simulink model "Comparison_Modulation_Techniques"  (R2021a)
settings: Solver=VariableStepAuto  StartTime=0.0  StopTime=10.0  RelTol=1e-3
libraries: commchan3 x4, commdigbbndpm3 x4, commsink2 x4, commrandsrc3 x3, commdigbbndfm2 x2, commdigbbndam3 x2, dspsrcs4 x1, dspquant2 x1
settings Model: Creator=Bharat Gunhalkar  LastModifiedBy=Bharat Gunhalkar

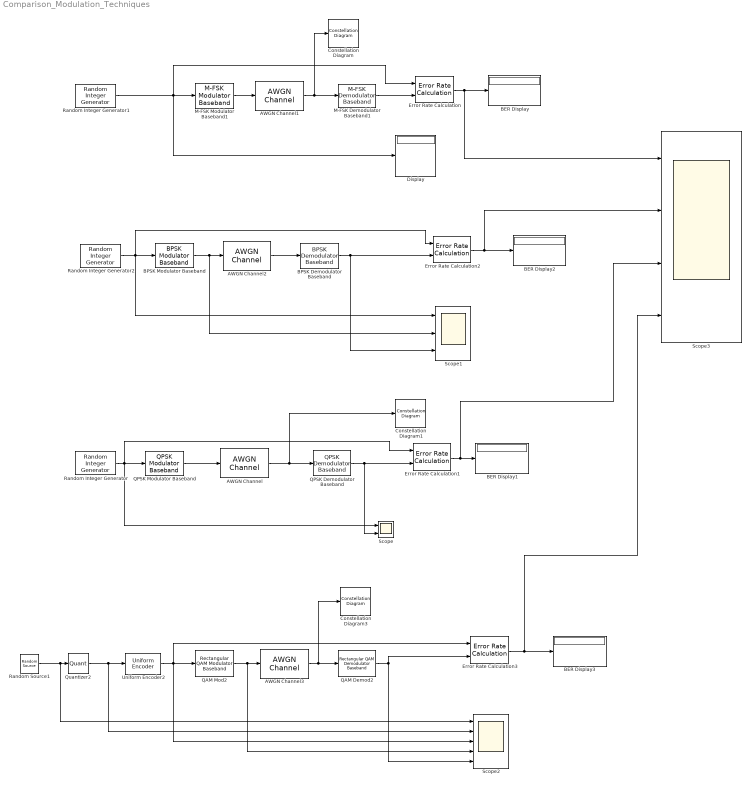
== system Comparison_Modulation_Techniques ==
  AWGN Channel : commchan3/AWGN Channel  InputProcessing=Columns as channels (frame based)  seed=67  noiseMode="Signal to noise ratio  (Eb/No)"  EbNodB=1  EsNodB=10  SNRdB=10  bitsPerSym=2  Ps=1  Tsym=1  variance=1
  AWGN Channel1 : commchan3/AWGN Channel  InputProcessing=Columns as channels (frame based)  seed=67  noiseMode="Signal to noise ratio  (Eb/No)"  EbNodB=1  EsNodB=10  SNRdB=10  bitsPerSym=1  Ps=1  Tsym=1  variance=1
  AWGN Channel2 : commchan3/AWGN Channel  InputProcessing=Columns as channels (frame based)  seed=67  noiseMode="Signal to noise ratio  (Eb/No)"  EbNodB=1  EsNodB=10  SNRdB=10  bitsPerSym=1  Ps=1  Tsym=1  variance=1
  AWGN Channel3 : commchan3/AWGN Channel  InputProcessing=Columns as channels (frame based)  seed=67  noiseMode="Signal to noise ratio  (Eb/No)"  EbNodB=1  EsNodB=10  SNRdB=10  bitsPerSym=1  Ps=1  Tsym=1  variance=1
  BER Display{,1..3} (4 alike) : Display
  BPSK Demodulator Baseband : commdigbbndpm3/BPSK Demodulator Baseband  DecType=Hard decision  VarSource=Dialog  Variance=1  Ph=0  outDtype=Inherit via internal rule  derotateFactorWordLen=16  derotateFactorDataTypeStr=Inherit: Same word length as input  derotateFactorLastDataTypeStr=Inherit: Same word length as input
  BPSK Modulator Baseband : commdigbbndpm3/BPSK Modulator Baseband  Ph=0  outDtype=double  outWordLen=16  outUDDataType=sfix(16)  outFracLenMode=Best precision  outFracLen=15  outDataTypeStr=double  outLastDataTypeStr=double
  Constellation Diagram : ConstellationDiagram
  Constellation Diagram1 : ConstellationDiagram
  Constellation Diagram3 : ConstellationDiagram
  Display : Display
  Error Rate Calculation{,1..3} (4 alike) : commsink2/Error Rate Calculation  N=0  st_delay=0  cp_mode=Entire frame  subframe=[]  PMode=Port  WsName=ErrorVec  RsMode2=off  stop=off  numErr=100  maxBits=1e6
  M-FSK Demodulator Baseband1 : commdigbbndfm2/M-FSK Demodulator Baseband  M=8  OutType=Integer  Dec=Gray  freqSep=6  numSamp=17  RateOptions=Enforce single-rate processing  outDataType=double
      settings: SourceProductBaseCode=CM
  M-FSK Modulator Baseband1 : commdigbbndfm2/M-FSK Modulator Baseband  M=8  InType=Integer  Enc=Gray  freqSep=6  phaseType=Continuous  numSamp=17  RateOptions=Enforce single-rate processing  outDataType=double
  QAM Demod2 : commdigbbndam3/Rectangular QAM Demodulator Baseband  M=16  OutType=Integer  DecType=Hard decision  VarSource=Dialog  Variance=1  Dec=Gray  Mapping=[0:15]  PowType=Min. distance between symbols  MinDist=2  AvgPow=1  PeakPow=1  Ph=0  outDtype1=Inherit via internal rule  outDtype2=Inherit via internal rule  derotateFactorWordLen=16  derotateFactorDataTypeStr=Inherit: Same word length as input  derotateFactorLastDataTypeStr=Inherit: Same word length as input  denormFactorWordLen=16  denormFactorDataTypeStr=Inherit: Same word length as input  denormFactorLastDataTypeStr=Inherit: Same word length as input  prodOutWordLen=32  prodOutOverflowMode=Wrap  prodOutRoundingMode=Floor  prodOutOvFlMode=off  prodOutOvFlModeLastStrValue=off  sumWordLen=32
  QAM Mod2 : commdigbbndam3/Rectangular QAM Modulator Baseband  M=16  InType=Integer  Enc=Gray  Mapping=[0:15]  PowType=Min. distance between symbols  MinDist=2  AvgPow=1  PeakPow=1  Ph=0  outDtype=double  outWordLen=16  outUDDataType=sfix(16)  outFracLenMode=Best precision  outFracLen=15  outDataTypeStr=double  outLastDataTypeStr=double
  QPSK Demodulator Baseband : commdigbbndpm3/QPSK Demodulator Baseband  OutType=Integer  DecType=Hard decision  VarSource=Dialog  Variance=1  Dec=Gray  Ph=pi/4  outDtype1=Inherit via internal rule  outDtype2=Inherit via internal rule  derotateFactorWordLen=16  derotateFactorDataTypeStr=Inherit: Same word length as input  derotateFactorLastDataTypeStr=Inherit: Same word length as input
  QPSK Modulator Baseband : commdigbbndpm3/QPSK Modulator Baseband  InType=Integer  Enc=Gray  Ph=pi/4  outDtype=double  outWordLen=16  outUDDataType=sfix(16)  outFracLenMode=Best precision  outFracLen=15  outDataTypeStr=double  outLastDataTypeStr=double
  Quantizer2 : Quantizer  QuantizationInterval=0.25  LinearizeAsGain=off
  Random Source1 : dspsrcs4/Random Source  SrcType=Uniform  NormMethod=Ziggurat  CltLength=12  MinVal=0  MaxVal=1  MeanVal=0  VarVal=1  RepMode=Not repeatable  rawSeed=1  IsInherit=off  SampMode=Discrete  SampTime=0.1  SampFrame=1  DataType=Single  OutComplex=Real  OutputFrames=off
  Random Integer Generator : commrandsrc3/Random Integer Generator  SetSize=4  SeedSource=Auto  Seed=0  SampleTime=1  SamplesPerFrame=1  OutputDataType=double  SimulateUsing=Interpreted execution
  Random Integer Generator1 : commrandsrc3/Random Integer Generator  SetSize=8  SeedSource=Auto  Seed=0  SampleTime=1  SamplesPerFrame=100  OutputDataType=double  SimulateUsing=Interpreted execution
  Random Integer Generator2 : commrandsrc3/Random Integer Generator  SetSize=2  SeedSource=Auto  Seed=0  SampleTime=0.1  SamplesPerFrame=1  OutputDataType=double  SimulateUsing=Interpreted execution
  Scope : Scope  NumInputPorts=2
  Scope1 : Scope  NumInputPorts=3
  Scope2 : Scope  NumInputPorts=5
  Scope3 : Scope  NumInputPorts=4
  Uniform Encoder2 : dspquant2/Uniform Encoder  peak=1  bits=4  otype=Unsigned integer
  wires:
  M-FSK Modulator Baseband1/1 -> AWGN Channel1/1
  Error Rate Calculation/1 -> Scope3/1, BER Display/1
  M-FSK Demodulator Baseband1/1 -> Error Rate Calculation/2
  AWGN Channel1/1 -> M-FSK Demodulator Baseband1/1, Constellation Diagram/1
  Random Integer Generator1/1 -> Display/1, Error Rate Calculation/1, M-FSK Modulator Baseband1/1
  AWGN Channel2/1 -> BPSK Demodulator Baseband/1
  Error Rate Calculation2/1 -> Scope3/2, BER Display2/1
  BPSK Demodulator Baseband/1 -> Error Rate Calculation2/2, Scope1/3
  Random Integer Generator2/1 -> Scope1/1, BPSK Modulator Baseband/1, Error Rate Calculation2/1
  BPSK Modulator Baseband/1 -> Scope1/2, AWGN Channel2/1
  Error Rate Calculation1/1 -> Scope3/3, BER Display1/1
  QPSK Demodulator Baseband/1 -> Error Rate Calculation1/2, Scope/2
  QPSK Modulator Baseband/1 -> AWGN Channel/1
  AWGN Channel/1 -> Constellation Diagram1/1, QPSK Demodulator Baseband/1
  Random Integer Generator/1 -> Scope/1, Error Rate Calculation1/1, QPSK Modulator Baseband/1
  AWGN Channel3/1 -> QAM Demod2/1, Constellation Diagram3/1
  Uniform Encoder2/1 -> QAM Mod2/1, Error Rate Calculation3/1, Scope2/3
  Quantizer2/1 -> Uniform Encoder2/1, Scope2/2
  Error Rate Calculation3/1 -> Scope3/4, BER Display3/1
  Random Source1/1 -> Scope2/1, Quantizer2/1
  QAM Mod2/1 -> AWGN Channel3/1, Scope2/4
  QAM Demod2/1 -> Error Rate Calculation3/2, Scope2/5
